simulink model "Appl_PaMemory_CtrlModel"  (R2018b)
settings: configuration reference "CodeConfig_10_ms" (kept outside this file)
undefined symbols (not defined in the file): CAL_PaMem_100MS, CAL_PaMem_90MS, D_ToleranceDistance, FALSE, TRUE
libraries: DareLib x89, simulink x1
(part 2 of 3)

== system Appl_PaMemory_CtrlModel/UpDataInputInfo/InputSignalProcess/HmiMessageDeal ==
  PaMem_IVI_FRSeatMemSet1 : Inport
  PaMem_IVI_FRSeatMemSet2 : Inport  Port=2
  PaMem_IVI_FRSeatMemSet3 : Inport  Port=3
  HmiDeal : Stateflow chart  TreatAsAtomicUnit=on
  SeatMemBtn : Outport
  wires:
  PaMem_IVI_FRSeatMemSet1/1 -> HmiDeal/1(PaMem_IVI_FLSeatMemSet1)
  PaMem_IVI_FRSeatMemSet2/1 -> HmiDeal/2(PaMem_IVI_FLSeatMemSet2)
  HmiDeal/1(SeatMemBtn) -> SeatMemBtn/1
  PaMem_IVI_FRSeatMemSet3/1 -> HmiDeal/3(PaMem_IVI_FLSeatMemSet3)

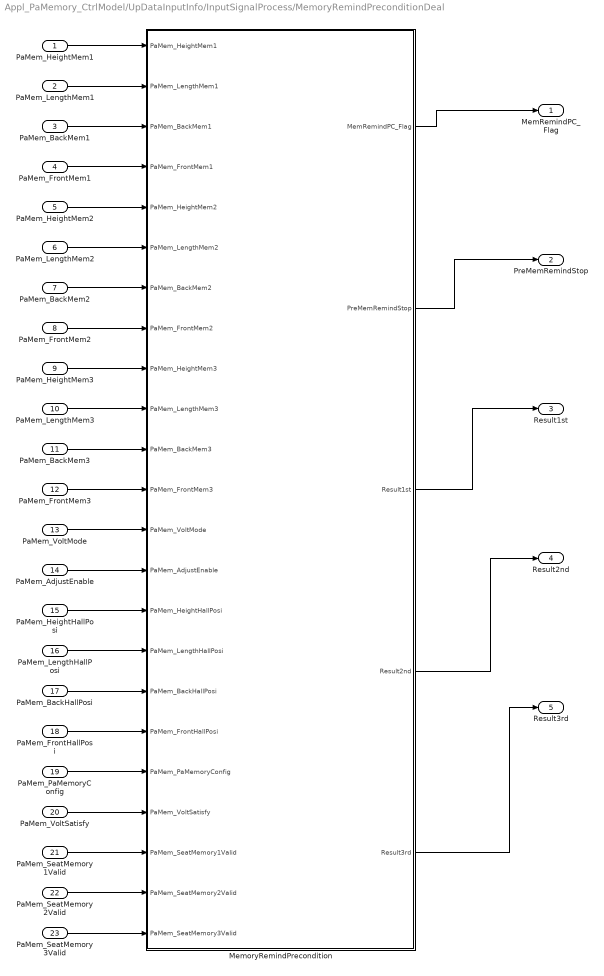
== system Appl_PaMemory_CtrlModel/UpDataInputInfo/InputSignalProcess/MemoryRemindPreconditionDeal ==
  PaMem_HeightMem1 : Inport
  PaMem_LengthMem1 : Inport  Port=2
  PaMem_BackMem1 : Inport  Port=3
  PaMem_FrontMem1 : Inport  Port=4
  PaMem_HeightMem2 : Inport  Port=5
  PaMem_LengthMem2 : Inport  Port=6
  PaMem_BackMem2 : Inport  Port=7
  PaMem_FrontMem2 : Inport  Port=8
  PaMem_HeightMem3 : Inport  Port=9
  PaMem_LengthMem3 : Inport  Port=10
  PaMem_BackMem3 : Inport  Port=11
  PaMem_FrontMem3 : Inport  Port=12
  PaMem_VoltMode : Inport  Port=13
  PaMem_AdjustEnable : Inport  Port=14
  PaMem_HeightHallPosi : Inport  Port=15
  PaMem_LengthHallPosi : Inport  Port=16
  PaMem_BackHallPosi : Inport  Port=17
  PaMem_FrontHallPosi : Inport  Port=18
  PaMem_PaMemoryConfig : Inport  Port=19
  PaMem_VoltSatisfy : Inport  Port=20
  PaMem_SeatMemory1Valid : Inport  Port=21
  PaMem_SeatMemory2Valid : Inport  Port=22
  PaMem_SeatMemory3Valid : Inport  Port=23
  MemoryRemindPrecondition : Stateflow chart  TreatAsAtomicUnit=on
  MemRemindPC_Flag : Outport
  PreMemRemindStop : Outport  Port=2
  Result1st : Outport  Port=3
  Result2nd : Outport  Port=4
  Result3rd : Outport  Port=5
  wires:
  PaMem_FrontMem3/1 -> MemoryRemindPrecondition/12(PaMem_FrontMem3)
  PaMem_VoltMode/1 -> MemoryRemindPrecondition/13(PaMem_VoltMode)
  PaMem_BackMem3/1 -> MemoryRemindPrecondition/11(PaMem_BackMem3)
  PaMem_LengthMem3/1 -> MemoryRemindPrecondition/10(PaMem_LengthMem3)
  PaMem_HeightMem3/1 -> MemoryRemindPrecondition/9(PaMem_HeightMem3)
  PaMem_FrontMem2/1 -> MemoryRemindPrecondition/8(PaMem_FrontMem2)
  PaMem_BackMem2/1 -> MemoryRemindPrecondition/7(PaMem_BackMem2)
  PaMem_LengthMem2/1 -> MemoryRemindPrecondition/6(PaMem_LengthMem2)
  PaMem_HeightMem2/1 -> MemoryRemindPrecondition/5(PaMem_HeightMem2)
  PaMem_FrontMem1/1 -> MemoryRemindPrecondition/4(PaMem_FrontMem1)
  PaMem_HeightMem1/1 -> MemoryRemindPrecondition/1(PaMem_HeightMem1)
  PaMem_BackMem1/1 -> MemoryRemindPrecondition/3(PaMem_BackMem1)
  PaMem_LengthMem1/1 -> MemoryRemindPrecondition/2(PaMem_LengthMem1)
  PaMem_AdjustEnable/1 -> MemoryRemindPrecondition/14(PaMem_AdjustEnable)
  PaMem_HeightHallPosi/1 -> MemoryRemindPrecondition/15(PaMem_HeightHallPosi)
  PaMem_LengthHallPosi/1 -> MemoryRemindPrecondition/16(PaMem_LengthHallPosi)
  PaMem_BackHallPosi/1 -> MemoryRemindPrecondition/17(PaMem_BackHallPosi)
  PaMem_FrontHallPosi/1 -> MemoryRemindPrecondition/18(PaMem_FrontHallPosi)
  MemoryRemindPrecondition/1(MemRemindPC_Flag) -> MemRemindPC_Flag/1
  MemoryRemindPrecondition/2(PreMemRemindStop) -> PreMemRemindStop/1
  MemoryRemindPrecondition/3(Result1st) -> Result1st/1
  MemoryRemindPrecondition/4(Result2nd) -> Result2nd/1
  MemoryRemindPrecondition/5(Result3rd) -> Result3rd/1
  PaMem_PaMemoryConfig/1 -> MemoryRemindPrecondition/19(PaMem_PaMemoryConfig)
  PaMem_VoltSatisfy/1 -> MemoryRemindPrecondition/20(PaMem_VoltSatisfy)
  PaMem_SeatMemory1Valid/1 -> MemoryRemindPrecondition/21(PaMem_SeatMemory1Valid)
  PaMem_SeatMemory2Valid/1 -> MemoryRemindPrecondition/22(PaMem_SeatMemory2Valid)
  PaMem_SeatMemory3Valid/1 -> MemoryRemindPrecondition/23(PaMem_SeatMemory3Valid)

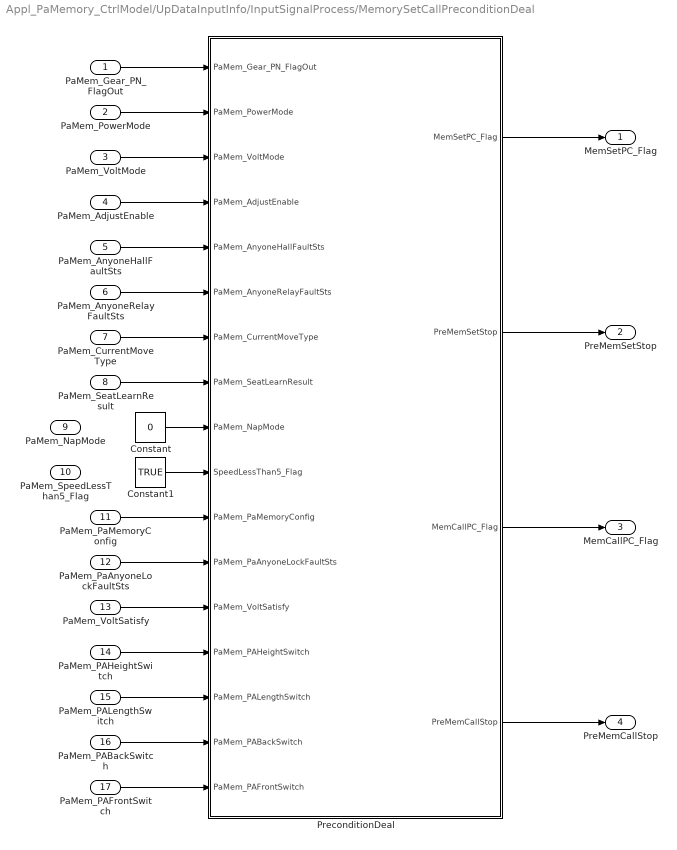
== system Appl_PaMemory_CtrlModel/UpDataInputInfo/InputSignalProcess/MemorySetCallPreconditionDeal ==
  PaMem_Gear_PN_FlagOut : Inport
  PaMem_PowerMode : Inport  Port=2
  PaMem_VoltMode : Inport  Port=3
  PaMem_AdjustEnable : Inport  Port=4
  PaMem_AnyoneHallFaultSts : Inport  Port=5
  PaMem_AnyoneRelayFaultSts : Inport  Port=6
  PaMem_CurrentMoveType : Inport  Port=7
  PaMem_SeatLearnResult : Inport  Port=8
  PaMem_NapMode : Inport  Port=9
  PaMem_SpeedLessThan5_Flag : Inport  Port=10
  PaMem_PaMemoryConfig : Inport  Port=11
  PaMem_PaAnyoneLockFaultSts : Inport  Port=12
  PaMem_VoltSatisfy : Inport  Port=13
  PaMem_PAHeightSwitch : Inport  Port=14
  PaMem_PALengthSwitch : Inport  Port=15
  PaMem_PABackSwitch : Inport  Port=16
  PaMem_PAFrontSwitch : Inport  Port=17
  Constant : Constant  Value=0  OutDataTypeStr=uint8
  Constant1 : Constant  Value=TRUE  OutDataTypeStr=uint8
  PreconditionDeal : Stateflow chart  TreatAsAtomicUnit=on
  MemSetPC_Flag : Outport
  PreMemSetStop : Outport  Port=2
  MemCallPC_Flag : Outport  Port=3
  PreMemCallStop : Outport  Port=4
  wires:
  PaMem_Gear_PN_FlagOut/1 -> PreconditionDeal/1(PaMem_Gear_PN_FlagOut)
  PaMem_PowerMode/1 -> PreconditionDeal/2(PaMem_PowerMode)
  PaMem_VoltMode/1 -> PreconditionDeal/3(PaMem_VoltMode)
  PaMem_AdjustEnable/1 -> PreconditionDeal/4(PaMem_AdjustEnable)
  PaMem_AnyoneHallFaultSts/1 -> PreconditionDeal/5(PaMem_AnyoneHallFaultSts)
  PaMem_CurrentMoveType/1 -> PreconditionDeal/7(PaMem_CurrentMoveType)
  PaMem_SeatLearnResult/1 -> PreconditionDeal/8(PaMem_SeatLearnResult)
  PaMem_AnyoneRelayFaultSts/1 -> PreconditionDeal/6(PaMem_AnyoneRelayFaultSts)
  PreconditionDeal/1(MemSetPC_Flag) -> MemSetPC_Flag/1
  PreconditionDeal/2(PreMemSetStop) -> PreMemSetStop/1
  PreconditionDeal/3(MemCallPC_Flag) -> MemCallPC_Flag/1
  PreconditionDeal/4(PreMemCallStop) -> PreMemCallStop/1
  PaMem_PaMemoryConfig/1 -> PreconditionDeal/11(PaMem_PaMemoryConfig)
  PaMem_PaAnyoneLockFaultSts/1 -> PreconditionDeal/12(PaMem_PaAnyoneLockFaultSts)
  Constant/1 -> PreconditionDeal/9(PaMem_NapMode)
  PaMem_VoltSatisfy/1 -> PreconditionDeal/13(PaMem_VoltSatisfy)
  PaMem_PAHeightSwitch/1 -> PreconditionDeal/14(PaMem_PAHeightSwitch)
  PaMem_PALengthSwitch/1 -> PreconditionDeal/15(PaMem_PALengthSwitch)
  PaMem_PABackSwitch/1 -> PreconditionDeal/16(PaMem_PABackSwitch)
  PaMem_PAFrontSwitch/1 -> PreconditionDeal/17(PaMem_PAFrontSwitch)
  Constant1/1 -> PreconditionDeal/10(SpeedLessThan5_Flag)

== system Appl_PaMemory_CtrlModel/LogicCtrl/LocalAdjustCtrl/MemorySetLogic/FirstPosiMemSetFunc/FirstPosiMemSetFunc/MemoryBack ==
  CurrentB : Inport
  f : TriggerPort  TriggerType=function-call  VariantControl=(inherit)
      settings: CopyFcn=Stateflow.SLINSF.SimulinkMan.removeBlockPreDeleteFcn  PreDeleteFcn=Stateflow.SLINSF.SimulinkMan.unsafePredeleteFcn
  WelcomeRunStatus : DareLib/Dare/setAPI_type  g_funcname=Srvl_SetMemIndexDataU16  g_param=EN_MemIndex_PaMem1_Back  g_type=uint16  g_size=-1
      settings: AttributesFormatString=%<g_funcname>  SourceProductName=Dare Library
  wires:
  CurrentB/1 -> WelcomeRunStatus/1

== system Appl_PaMemory_CtrlModel/LogicCtrl/LocalAdjustCtrl/MemorySetLogic/FirstPosiMemSetFunc/FirstPosiMemSetFunc/MemoryFront ==
  CurrentF : Inport
  f : TriggerPort  TriggerType=function-call  VariantControl=(inherit)
      settings: CopyFcn=Stateflow.SLINSF.SimulinkMan.removeBlockPreDeleteFcn  PreDeleteFcn=Stateflow.SLINSF.SimulinkMan.unsafePredeleteFcn
  WelcomeRunStatus : DareLib/Dare/setAPI_type  g_funcname=Srvl_SetMemIndexDataU16  g_param=EN_MemIndex_PaMem1_Front  g_type=uint16  g_size=-1
      settings: AttributesFormatString=%<g_funcname>  SourceProductName=Dare Library
  wires:
  CurrentF/1 -> WelcomeRunStatus/1

== system Appl_PaMemory_CtrlModel/LogicCtrl/LocalAdjustCtrl/MemorySetLogic/FirstPosiMemSetFunc/FirstPosiMemSetFunc/MemoryHight ==
  CurrentH : Inport
  f : TriggerPort  TriggerType=function-call  VariantControl=(inherit)
      settings: CopyFcn=Stateflow.SLINSF.SimulinkMan.removeBlockPreDeleteFcn  PreDeleteFcn=Stateflow.SLINSF.SimulinkMan.unsafePredeleteFcn
  WelcomeRunStatus : DareLib/Dare/setAPI_type  g_funcname=Srvl_SetMemIndexDataU16  g_param=EN_MemIndex_PaMem1_Height  g_type=uint16  g_size=-1
      settings: AttributesFormatString=%<g_funcname>  SourceProductName=Dare Library
  wires:
  CurrentH/1 -> WelcomeRunStatus/1

== system Appl_PaMemory_CtrlModel/LogicCtrl/LocalAdjustCtrl/MemorySetLogic/FirstPosiMemSetFunc/FirstPosiMemSetFunc/MemoryLength ==
  CurrentL : Inport
  f : TriggerPort  TriggerType=function-call  VariantControl=(inherit)
      settings: CopyFcn=Stateflow.SLINSF.SimulinkMan.removeBlockPreDeleteFcn  PreDeleteFcn=Stateflow.SLINSF.SimulinkMan.unsafePredeleteFcn
  WelcomeRunStatus : DareLib/Dare/setAPI_type  g_funcname=Srvl_SetMemIndexDataU16  g_param=EN_MemIndex_PaMem1_Length  g_type=uint16  g_size=-1
      settings: AttributesFormatString=%<g_funcname>  SourceProductName=Dare Library
  wires:
  CurrentL/1 -> WelcomeRunStatus/1

== system Appl_PaMemory_CtrlModel/LogicCtrl/LocalAdjustCtrl/MemorySetLogic/FirstPosiMemSetFunc/FirstPosiMemSetFunc/MemoryValid ==
  Sts : Inport
  f : TriggerPort  TriggerType=function-call  VariantControl=(inherit)
      settings: CopyFcn=Stateflow.SLINSF.SimulinkMan.removeBlockPreDeleteFcn  PreDeleteFcn=Stateflow.SLINSF.SimulinkMan.unsafePredeleteFcn
  WelcomeRunStatus : DareLib/Dare/setAPI_type  g_funcname=Srvl_SetMemIndexDataU8  g_param=EN_MemIndex_PaMem1_ValidFlag  g_type=uint16  g_size=-1
      settings: AttributesFormatString=%<g_funcname>  SourceProductName=Dare Library
  wires:
  Sts/1 -> WelcomeRunStatus/1

== system Appl_PaMemory_CtrlModel/LogicCtrl/LocalAdjustCtrl/MemorySetLogic/SecondPosiMemSetFunc/SecondPosiMemSetFunc/MemoryBack ==
  CurrentB : Inport
  f : TriggerPort  TriggerType=function-call  VariantControl=(inherit)
      settings: CopyFcn=Stateflow.SLINSF.SimulinkMan.removeBlockPreDeleteFcn  PreDeleteFcn=Stateflow.SLINSF.SimulinkMan.unsafePredeleteFcn
  WelcomeRunStatus : DareLib/Dare/setAPI_type  g_funcname=Srvl_SetMemIndexDataU16  g_param=EN_MemIndex_PaMem2_Back  g_type=uint16  g_size=-1
      settings: AttributesFormatString=%<g_funcname>  SourceProductName=Dare Library
  wires:
  CurrentB/1 -> WelcomeRunStatus/1

== system Appl_PaMemory_CtrlModel/LogicCtrl/LocalAdjustCtrl/MemorySetLogic/SecondPosiMemSetFunc/SecondPosiMemSetFunc/MemoryFront ==
  CurrentF : Inport
  f : TriggerPort  TriggerType=function-call  VariantControl=(inherit)
      settings: CopyFcn=Stateflow.SLINSF.SimulinkMan.removeBlockPreDeleteFcn  PreDeleteFcn=Stateflow.SLINSF.SimulinkMan.unsafePredeleteFcn
  WelcomeRunStatus : DareLib/Dare/setAPI_type  g_funcname=Srvl_SetMemIndexDataU16  g_param=EN_MemIndex_PaMem2_Front  g_type=uint16  g_size=-1
      settings: AttributesFormatString=%<g_funcname>  SourceProductName=Dare Library
  wires:
  CurrentF/1 -> WelcomeRunStatus/1

== system Appl_PaMemory_CtrlModel/LogicCtrl/LocalAdjustCtrl/MemorySetLogic/SecondPosiMemSetFunc/SecondPosiMemSetFunc/MemoryHight ==
  CurrentH : Inport
  f : TriggerPort  TriggerType=function-call  VariantControl=(inherit)
      settings: CopyFcn=Stateflow.SLINSF.SimulinkMan.removeBlockPreDeleteFcn  PreDeleteFcn=Stateflow.SLINSF.SimulinkMan.unsafePredeleteFcn
  WelcomeRunStatus : DareLib/Dare/setAPI_type  g_funcname=Srvl_SetMemIndexDataU16  g_param=EN_MemIndex_PaMem2_Height  g_type=uint16  g_size=-1
      settings: AttributesFormatString=%<g_funcname>  SourceProductName=Dare Library
  wires:
  CurrentH/1 -> WelcomeRunStatus/1

== system Appl_PaMemory_CtrlModel/LogicCtrl/LocalAdjustCtrl/MemorySetLogic/SecondPosiMemSetFunc/SecondPosiMemSetFunc/MemoryLength ==
  CurrentL : Inport
  f : TriggerPort  TriggerType=function-call  VariantControl=(inherit)
      settings: CopyFcn=Stateflow.SLINSF.SimulinkMan.removeBlockPreDeleteFcn  PreDeleteFcn=Stateflow.SLINSF.SimulinkMan.unsafePredeleteFcn
  WelcomeRunStatus : DareLib/Dare/setAPI_type  g_funcname=Srvl_SetMemIndexDataU16  g_param=EN_MemIndex_PaMem2_Length  g_type=uint16  g_size=-1
      settings: AttributesFormatString=%<g_funcname>  SourceProductName=Dare Library
  wires:
  CurrentL/1 -> WelcomeRunStatus/1

== system Appl_PaMemory_CtrlModel/LogicCtrl/LocalAdjustCtrl/MemorySetLogic/SecondPosiMemSetFunc/SecondPosiMemSetFunc/MemoryValid ==
  Sts : Inport
  f : TriggerPort  TriggerType=function-call  VariantControl=(inherit)
      settings: CopyFcn=Stateflow.SLINSF.SimulinkMan.removeBlockPreDeleteFcn  PreDeleteFcn=Stateflow.SLINSF.SimulinkMan.unsafePredeleteFcn
  WelcomeRunStatus : DareLib/Dare/setAPI_type  g_funcname=Srvl_SetMemIndexDataU8  g_param=EN_MemIndex_PaMem2_ValidFlag  g_type=uint16  g_size=-1
      settings: AttributesFormatString=%<g_funcname>  SourceProductName=Dare Library
  wires:
  Sts/1 -> WelcomeRunStatus/1

== system Appl_PaMemory_CtrlModel/LogicCtrl/LocalAdjustCtrl/MemorySetLogic/ThirdPosiMemSetFunc/ThirdPosiMemSetFunc/MemoryBack ==
  CurrentB : Inport
  f : TriggerPort  TriggerType=function-call  VariantControl=(inherit)
      settings: CopyFcn=Stateflow.SLINSF.SimulinkMan.removeBlockPreDeleteFcn  PreDeleteFcn=Stateflow.SLINSF.SimulinkMan.unsafePredeleteFcn
  WelcomeRunStatus : DareLib/Dare/setAPI_type  g_funcname=Srvl_SetMemIndexDataU16  g_param=EN_MemIndex_PaMem3_Back  g_type=uint16  g_size=-1
      settings: AttributesFormatString=%<g_funcname>  SourceProductName=Dare Library
  wires:
  CurrentB/1 -> WelcomeRunStatus/1

== system Appl_PaMemory_CtrlModel/LogicCtrl/LocalAdjustCtrl/MemorySetLogic/ThirdPosiMemSetFunc/ThirdPosiMemSetFunc/MemoryFront ==
  CurrentF : Inport
  f : TriggerPort  TriggerType=function-call  VariantControl=(inherit)
      settings: CopyFcn=Stateflow.SLINSF.SimulinkMan.removeBlockPreDeleteFcn  PreDeleteFcn=Stateflow.SLINSF.SimulinkMan.unsafePredeleteFcn
  WelcomeRunStatus : DareLib/Dare/setAPI_type  g_funcname=Srvl_SetMemIndexDataU16  g_param=EN_MemIndex_PaMem3_Front  g_type=uint16  g_size=-1
      settings: AttributesFormatString=%<g_funcname>  SourceProductName=Dare Library
  wires:
  CurrentF/1 -> WelcomeRunStatus/1

== system Appl_PaMemory_CtrlModel/LogicCtrl/LocalAdjustCtrl/MemorySetLogic/ThirdPosiMemSetFunc/ThirdPosiMemSetFunc/MemoryHight ==
  CurrentH : Inport
  f : TriggerPort  TriggerType=function-call  VariantControl=(inherit)
      settings: CopyFcn=Stateflow.SLINSF.SimulinkMan.removeBlockPreDeleteFcn  PreDeleteFcn=Stateflow.SLINSF.SimulinkMan.unsafePredeleteFcn
  WelcomeRunStatus : DareLib/Dare/setAPI_type  g_funcname=Srvl_SetMemIndexDataU16  g_param=EN_MemIndex_PaMem3_Height  g_type=uint16  g_size=-1
      settings: AttributesFormatString=%<g_funcname>  SourceProductName=Dare Library
  wires:
  CurrentH/1 -> WelcomeRunStatus/1

== system Appl_PaMemory_CtrlModel/LogicCtrl/LocalAdjustCtrl/MemorySetLogic/ThirdPosiMemSetFunc/ThirdPosiMemSetFunc/MemoryLength ==
  CurrentL : Inport
  f : TriggerPort  TriggerType=function-call  VariantControl=(inherit)
      settings: CopyFcn=Stateflow.SLINSF.SimulinkMan.removeBlockPreDeleteFcn  PreDeleteFcn=Stateflow.SLINSF.SimulinkMan.unsafePredeleteFcn
  WelcomeRunStatus : DareLib/Dare/setAPI_type  g_funcname=Srvl_SetMemIndexDataU16  g_param=EN_MemIndex_PaMem3_Length  g_type=uint16  g_size=-1
      settings: AttributesFormatString=%<g_funcname>  SourceProductName=Dare Library
  wires:
  CurrentL/1 -> WelcomeRunStatus/1

== system Appl_PaMemory_CtrlModel/LogicCtrl/LocalAdjustCtrl/MemorySetLogic/ThirdPosiMemSetFunc/ThirdPosiMemSetFunc/MemoryValid ==
  Sts : Inport
  f : TriggerPort  TriggerType=function-call  VariantControl=(inherit)
      settings: CopyFcn=Stateflow.SLINSF.SimulinkMan.removeBlockPreDeleteFcn  PreDeleteFcn=Stateflow.SLINSF.SimulinkMan.unsafePredeleteFcn
  WelcomeRunStatus : DareLib/Dare/setAPI_type  g_funcname=Srvl_SetMemIndexDataU8  g_param=EN_MemIndex_PaMem3_ValidFlag  g_type=uint16  g_size=-1
      settings: AttributesFormatString=%<g_funcname>  SourceProductName=Dare Library
  wires:
  Sts/1 -> WelcomeRunStatus/1

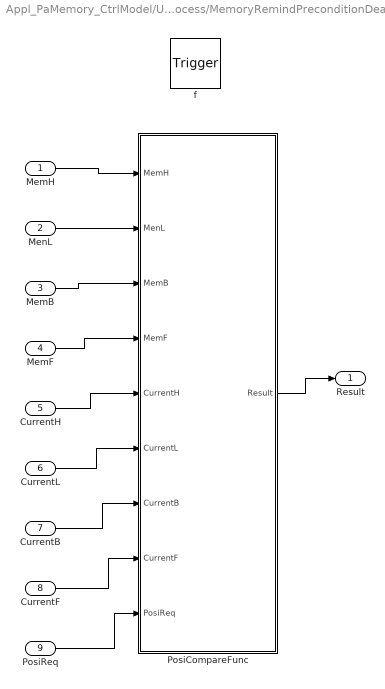
== system Appl_PaMemory_CtrlModel/UpDataInputInfo/InputSignalProcess/MemoryRemindPreconditionDeal/MemoryRemindPrecondition/PosiCompareFunc ==
  MemH : Inport
  MenL : Inport  Port=2
  MemB : Inport  Port=3
  MemF : Inport  Port=4
  CurrentH : Inport  Port=5
  CurrentL : Inport  Port=6
  CurrentB : Inport  Port=7
  CurrentF : Inport  Port=8
  PosiReq : Inport  Port=9
  f : TriggerPort  TriggerType=function-call  VariantControl=(inherit)
      settings: CopyFcn=Stateflow.SLINSF.SimulinkMan.removeBlockPreDeleteFcn  PreDeleteFcn=Stateflow.SLINSF.SimulinkMan.unsafePredeleteFcn
  PosiCompareFunc : Stateflow chart  TreatAsAtomicUnit=on
  "Result " : Outport
  wires:
  MemB/1 -> PosiCompareFunc/3(MemB)
  MemF/1 -> PosiCompareFunc/4(MemF)
  CurrentH/1 -> PosiCompareFunc/5(CurrentH)
  MenL/1 -> PosiCompareFunc/2(MenL)
  CurrentL/1 -> PosiCompareFunc/6(CurrentL)
  MemH/1 -> PosiCompareFunc/1(MemH)
  CurrentB/1 -> PosiCompareFunc/7(CurrentB)
  CurrentF/1 -> PosiCompareFunc/8(CurrentF)
  PosiCompareFunc/1(Result) -> "Result "/1
  PosiReq/1 -> PosiCompareFunc/9(PosiReq)

== stateflow chart Appl_PaMemory_CtrlModel/UpDataInputInfo/InputSignalProcess/CallMemDeal/CallMemory ==
  state NoneMemoryCall
    en:
    MemoryHeightPosi = 0;
    MemoryLengthPosi = 0;
    MemoryBackPosi = 0;
    MemoryFrontPosi = 0;
    MemoryValid = FALSE;
  state AcquireMemory2ndPosi
    en:
    MemoryHeightPosi = PaMem_HeightMem2;
    MemoryLengthPosi = PaMem_LengthMem2;
    MemoryBackPosi = PaMem_BackMem2;
    MemoryFrontPosi = PaMem_FrontMem2;
    MemoryValid = PaMem_SeatMemory2Valid;
  state AcquireMemory1stPosi
    en:
    MemoryHeightPosi = PaMem_HeightMem1;
    MemoryLengthPosi = PaMem_LengthMem1;
    MemoryBackPosi = PaMem_BackMem1;
    MemoryFrontPosi = PaMem_FrontMem1;
    MemoryValid = PaMem_SeatMemory1Valid;
  state AcquireMemory3rdPosi
    en:
    MemoryHeightPosi = PaMem_HeightMem3;
    MemoryLengthPosi = PaMem_LengthMem3;
    MemoryBackPosi = PaMem_BackMem3;
    MemoryFrontPosi = PaMem_FrontMem3;
    MemoryValid = PaMem_SeatMemory3Valid;
  (default) -> NoneMemoryCall
  NoneMemoryCall -> AcquireMemory1stPosi [order 1] : /* 调用位置1 */
      | [SeatMemBtn == enMemBtn.EN_MemBtn_Call1]
  AcquireMemory1stPosi -> NoneMemoryCall [order 1] : /* 无调用 */
      | [SeatMemBtn != enMemBtn.EN_MemBtn_Call1 ...
      | && SeatMemBtn != enMemBtn.EN_MemBtn_Call2 ...
      | && SeatMemBtn != enMemBtn.EN_MemBtn_Call3]
  NoneMemoryCall -> AcquireMemory2ndPosi [order 2] : /* 调用位置2 */
      | [SeatMemBtn == enMemBtn.EN_MemBtn_Call2]
  AcquireMemory2ndPosi -> NoneMemoryCall [order 1] : /* 无调用 */
      | [SeatMemBtn != enMemBtn.EN_MemBtn_Call1 ...
      | && SeatMemBtn != enMemBtn.EN_MemBtn_Call2 ...
      | && SeatMemBtn != enMemBtn.EN_MemBtn_Call3]
  NoneMemoryCall -> AcquireMemory3rdPosi [order 3] : /* 调用位置3 */
      | [SeatMemBtn == enMemBtn.EN_MemBtn_Call3]
  AcquireMemory3rdPosi -> NoneMemoryCall [order 1] : /* 无调用 */
      | [SeatMemBtn != enMemBtn.EN_MemBtn_Call1 ...
      | && SeatMemBtn != enMemBtn.EN_MemBtn_Call2 ...
      | && SeatMemBtn != enMemBtn.EN_MemBtn_Call3]
  AcquireMemory1stPosi -> AcquireMemory2ndPosi [order 3] : /* 调用位置2 */
      | [SeatMemBtn == enMemBtn.EN_MemBtn_Call2]
  AcquireMemory3rdPosi -> AcquireMemory2ndPosi [order 3] : /* 调用位置2 */
      | [SeatMemBtn == enMemBtn.EN_MemBtn_Call2]
  AcquireMemory2ndPosi -> AcquireMemory3rdPosi [order 3] : /* 调用位置3 */
      | [SeatMemBtn == enMemBtn.EN_MemBtn_Call3]
  AcquireMemory2ndPosi -> AcquireMemory1stPosi [order 2] : /* 调用位置1 */
      | [SeatMemBtn == enMemBtn.EN_MemBtn_Call1]
  AcquireMemory1stPosi -> AcquireMemory3rdPosi [order 2] : /* 调用位置3 */
      | [SeatMemBtn == enMemBtn.EN_MemBtn_Call3]
  AcquireMemory3rdPosi -> AcquireMemory1stPosi [order 2] : /* 调用位置1 */
      | [SeatMemBtn == enMemBtn.EN_MemBtn_Call1]
  data: PaMem_HeightMem1 input; MemoryHeightPosi output uint16; MemoryLengthPosi output uint16; MemoryBackPosi output uint16; MemoryFrontPosi output uint16; MemoryValid output uint8; PaMem_LengthMem1 input; PaMem_BackMem1 input; PaMem_FrontMem1 input; PaMem_HeightMem2 input; PaMem_LengthMem2 input; PaMem_BackMem2 input; PaMem_FrontMem2 input; PaMem_HeightMem3 input; PaMem_LengthMem3 input; PaMem_BackMem3 input; PaMem_FrontMem3 input; SeatMemBtn input; TRUE parameter; FALSE parameter; PaMem_SeatMemory1Valid input; PaMem_SeatMemory2Valid input; PaMem_SeatMemory3Valid input

== stateflow chart Appl_PaMemory_CtrlModel/UpDataInputInfo/InputSignalProcess/MemoryRemindPreconditionDeal/MemoryRemindPrecondition ==
  state Result = PosiCompareFunc(MemH,MenL,MemB,MemF,CurrentH,CurrentL,CurrentB,CurrentF,PosiReq) [function]
  state CompareCurrentAndMemoryPosi [parallel]
    du:
    Result1st = PosiCompareFunc(0,PaMem_LengthMem1,PaMem_BackMem1,0,0,PaMem_LengthHallPosi,PaMem_BackHallPosi,0,PaMem_SeatMemory1Valid);
    Result2nd = PosiCompareFunc(0,PaMem_LengthMem2,PaMem_BackMem2,0,0,PaMem_LengthHallPosi,PaMem_BackHallPosi,0,PaMem_SeatMemory2Valid);
    Result3rd = PosiCompareFunc(0,PaMem_LengthMem3,PaMem_BackMem3,0,0,PaMem_LengthHallPosi,PaMem_BackHallPosi,0,PaMem_SeatMemory3Valid);
    settings: executionOrder=1
  state MemoryRemindPreconditionDeal [parallel]
    settings: executionOrder=2
    state PreconditionNotSatisfied
      en:
      MemRemindPC_Flag = FALSE;
    state PreconditionSatisfied
      en:
      MemRemindPC_Flag = TRUE;
    (default) -> PreconditionNotSatisfied
    PreconditionNotSatisfied -> PreconditionSatisfied : /*记忆功能使能 == 0x1:TRUE
        | && 记忆提示功能使能 == 0x1:Enable
        | && 电压模式 == 正常
        | /PreMemRemindStop = 0x0:enNone;*/
        | [PaMem_AdjustEnable == TRUE ...
        | && PaMem_PaMemoryConfig == TRUE ...
        | && PaMem_VoltSatisfy == TRUE ...
        | && PaMem_VoltMode == enFinalPowerMode.EN_NORMAL_VOLT]
        | /PreMemRemindStop = enMemStopCause.EN_MemStop_NULL;
    PreconditionSatisfied -> PreconditionNotSatisfied [order 1] : /*F101记忆功能 != 0x1:TRUE
        | || 记忆提示功能配置 != 0x1:Enable
        | /PreMemRemindStop = 0xA:enConfigError;*/
        | [PaMem_AdjustEnable != TRUE || PaMem_PaMemoryConfig != TRUE]
        | /PreMemRemindStop = enMemStopCause.EN_MemStop_ConfigError;
    PreconditionSatisfied -> PreconditionNotSatisfied [order 2] : /*电压模式 != 正常
        | /PreMemRemindStop = 0xE:enVoltageError;*/
        | [PaMem_VoltMode != enFinalPowerMode.EN_NORMAL_VOLT ...
        | || PaMem_VoltSatisfy != TRUE]
        | /PreMemRemindStop = enMemStopCause.EN_MemStop_VoltageErr;
  data: MemH function_input; MenL function_input; MemB function_input; MemF function_input; CurrentH function_input; CurrentL function_input; CurrentB function_input; CurrentF function_input; Result function_output; PosiReq function_input; PaMem_HeightMem1 input; PaMem_LengthMem1 input; PaMem_BackMem1 input; PaMem_FrontMem1 input; PaMem_HeightMem2 input; PaMem_LengthMem2 input; PaMem_BackMem2 input; PaMem_FrontMem2 input; PaMem_HeightMem3 input; PaMem_LengthMem3 input; PaMem_BackMem3 input; PaMem_FrontMem3 input; PaMem_VoltMode input; TRUE parameter; PaMem_AdjustEnable input; FALSE parameter; MemRemindPC_Flag output uint8; PreMemRemindStop output Enum: enMemStopCause; Result1st output uint8; Result2nd output uint8; Result3rd output uint8; PaMem_HeightHallPosi input; PaMem_LengthHallPosi input; PaMem_BackHallPosi input; PaMem_FrontHallPosi input; PaMem_PaMemoryConfig input; PaMem_VoltSatisfy input; PaMem_SeatMemory1Valid input; PaMem_SeatMemory2Valid input; PaMem_SeatMemory3Valid input

== stateflow chart Appl_PaMemory_CtrlModel/LogicCtrl/LocalAdjustCtrl/MemorySetLogic ==
  state FirstPosiMemSetFunc(SeatMemCfg,CurrentH,CurrentL,CurrentB,CurrentF) [function]
  state MemorySetInactive
    en:
    FRSeatMemSetSts = enMemSetFb.EN_MemSetFb_NULL;
    MsgSendFinishedFlag = FALSE;
  state SecondPosiMemSetFunc(SeatMemCfg,CurrentH,CurrentL,CurrentB,CurrentF) [function]
  state MemorySetActive
    state Wait
      (default) -> (junction 127)
      Wait -> (junction 127) [order 1]
      (junction 127) -> (junction 30)
      (junction 30) -> (junction 122) [order 1] : /*初始前置条件不符合*/
          | [MemSetPC_Flag == FALSE]
      (junction 30) -> (junction 33) [order 2]
      (junction 122) -> (junction 124) : {WaitTimer = 0;}
      (junction 33) -> (junction 35) [order 1] : /*记忆设置1*/
          | [SeatMemBtn == enMemBtn.EN_MemBtn_Set1]
      (junction 33) -> (junction 39) [order 2]
      (junction 35) -> (junction 37) : {FRTempSeatMemSetSts = enMemSetFb.EN_MemSetFb_S1;
          | FirstPosiMemSetFunc(PaMem_AdjustEnable,PaMem_HeightHallPosi,PaMem_LengthHallPosi,PaMem_BackHallPosi,PaMem_FrontHallPosi);}
      (junction 37) -> (junction 39)
      (junction 39) -> (junction 42)
      (junction 42) -> (junction 44) [order 1] : /*记忆设置2*/
          | [SeatMemBtn == enMemBtn.EN_MemBtn_Set2]
      (junction 42) -> (junction 48) [order 2]
      (junction 44) -> (junction 46) : {FRTempSeatMemSetSts = enMemSetFb.EN_MemSetFb_S2;
          | SecondPosiMemSetFunc(PaMem_AdjustEnable,PaMem_HeightHallPosi,PaMem_LengthHallPosi,PaMem_BackHallPosi,PaMem_FrontHallPosi);}
      (junction 46) -> (junction 48)
      (junction 48) -> (junction 51)
      (junction 51) -> (junction 53) [order 1] : /*记忆设置3*/
          | [SeatMemBtn == enMemBtn.EN_MemBtn_Set3]
      (junction 51) -> (junction 57) [order 2]
      (junction 53) -> (junction 55) : {FRTempSeatMemSetSts = enMemSetFb.EN_MemSetFb_S3;
          | ThirdPosiMemSetFunc(PaMem_AdjustEnable,PaMem_HeightHallPosi,PaMem_LengthHallPosi,PaMem_BackHallPosi,PaMem_FrontHallPosi);}
      (junction 55) -> (junction 57)
      (junction 57) -> (junction 60) : {FRSeatMemSetSts = enMemSetFb.EN_MemSetFb_NULL;}
      (junction 60) -> (junction 62)
      (junction 62) -> (junction 64) [order 1] : /*使用延时代替EEPROM操作结果*/
          | [WaitTimer < CAL_PaMem_100MS]
      (junction 62) -> (junction 68) [order 2] : {WaitTimer = CAL_PaMem_100MS;}
      (junction 64) -> (junction 66) : {WaitTimer++ ;}
      (junction 66) -> (junction 68)
      (junction 124) -> (junction 66)
      (junction 68) -> (junction 72)
    state Succeed
      en:
      FRSeatMemSetSts = FRTempSeatMemSetSts;
      WaitTimer = 0;
      WaitTimeCnt = 0;
      SetCanSendMemStsAndMsg(FRSeatMemSetSts);
      SetCanSendEvent(0x3B2);
      du:
      WaitTimeCnt += 1;
    state Fail
      en:
      FRSeatMemSetSts = enMemSetFb.EN_MemSetFb_Fail;
      WaitTimer = 0;
      WaitTimeCnt = 0;
      SetCanSendMemStsAndMsg(FRSeatMemSetSts);
      SetCanSendEvent(0x3B2);
      du:
      WaitTimeCnt += 1;
    note: /*如果服务层没有CAN反馈标志，使用延时90ms(20ms/5帧)*/
    state MessageSendFinish
      en:
      MsgSendFinishedFlag = TRUE;
      FRSeatMemSetSts = enMemSetFb.EN_MemSetFb_NULL;
    (default) -> Wait
    Wait -> Succeed [order 2] : /*存储结束*/
        | [WaitTimer >= CAL_PaMem_100MS]
    Wait -> Fail [order 1] : /*前置条件不符合*/
        | [MemSetPC_Flag == FALSE]
        | /MemSetStopReason = PreMemSetStop;
    Wait -> Fail [commented out] : /*记忆存储失败，如果无此接口，删除*/
    Succeed -> MessageSendFinish : /*Srvl_CAN反馈报文发送完成 || 延时90ms*/
        | [WaitTimeCnt >= CAL_PaMem_90MS || GetCanSendEvent() == TRUE]
    Fail -> MessageSendFinish : /*Srvl_CAN反馈报文发送完成 || 延时90ms*/
        | [WaitTimeCnt >= CAL_PaMem_90MS || GetCanSendEvent() == TRUE]
  state ThirdPosiMemSetFunc(SeatMemCfg,CurrentH,CurrentL,CurrentB,CurrentF) [function]
  state SetCanSendEvent(In1) [function]
  state Out1 = GetCanSendEvent [function]
  state SetCanSendMemStsAndMsg(In1) [function]
  (default) -> MemorySetInactive
  MemorySetInactive -> MemorySetActive [order 1] : /*SeatMemBtn变为MemorizeButton1*/
      | [hasChangedTo(SeatMemBtn,enMemBtn.EN_MemBtn_Set1)]
  MemorySetInactive -> MemorySetActive [order 2] : /*SeatMemBtn变为MemorizeButton2*/
      | [hasChangedTo(SeatMemBtn,enMemBtn.EN_MemBtn_Set2)]
  MemorySetInactive -> MemorySetActive [order 3] : /*SeatMemBtn变为MemorizeButton3*/
      | [hasChangedTo(SeatMemBtn,enMemBtn.EN_MemBtn_Set3)]
  MemorySetActive -> MemorySetInactive : [MsgSendFinishedFlag == TRUE]
  data: SeatMemCfg function_input; CurrentH function_input; CurrentL function_input; CurrentB function_input; CurrentF function_input; SeatMemCfg function_input; CurrentH function_input; CurrentL function_input; CurrentB function_input; CurrentF function_input; SeatMemCfg function_input; CurrentH function_input; CurrentL function_input; CurrentB function_input; CurrentF function_input; In1 function_input; Out1 function_output; In1 function_input; FRSeatMemSetSts output Enum: enMemSetFb; MsgSendFinishedFlag local uint8; TRUE parameter; FALSE parameter; SeatMemBtn input; PaMem_HeightHallPosi input; PaMem_LengthHallPosi input; PaMem_BackHallPosi input; PaMem_FrontHallPosi input; MemSetPC_Flag input; WaitTimer local uint8; CAL_PaMem_100MS parameter; PreMemSetStop input; MemSetStopReason output Enum: enMemStopCause; FRTempSeatMemSetSts local Enum: enMemSetFb; PaMem_AdjustEnable input; CAL_PaMem_90MS parameter; WaitTimeCnt local uint16

== stateflow chart Appl_PaMemory_CtrlModel/UpDataInputInfo/InputSignalProcess/MemoryRemindPreconditionDeal/MemoryRemindPrecondition/PosiCompareFunc/PosiCompareFunc ==
  (default) -> (junction 15)
  (junction 15) -> (junction 30) [order 1] : /* 没有记忆位置 */
      | [PosiReq == FALSE]
  (junction 15) -> (junction 17) [order 2]
  (junction 30) -> (junction 34) : {Result = 2;}
  (junction 17) -> (junction 19) [order 1] : /* 当前位置在记忆位置范围内 */
      | [CurrentH <= MemH + D_ToleranceDistance ...
      | && MemH <= CurrentH  + D_ToleranceDistance ...
      | && CurrentL <= MenL + D_ToleranceDistance ...
      | && MenL <= CurrentL  + D_ToleranceDistance ...
      | && CurrentB <= MemB + D_ToleranceDistance ...
      | && MemB <= CurrentB  + D_ToleranceDistance ...
      | && CurrentF <= MemF + D_ToleranceDistance ...
      | && MemF <= CurrentF  + D_ToleranceDistance]
  (junction 17) -> (junction 23) [order 2] : {Result = FALSE;}
  (junction 19) -> (junction 21) : {Result = TRUE;}
  (junction 21) -> (junction 23)
  (junction 34) -> (junction 21)
  (junction 23) -> (junction 26)
  data: MemH input uint16; MenL input uint16; MemB input uint16; MemF input uint16; CurrentH input uint16; CurrentL input uint16; CurrentB input uint16; CurrentF input uint16; Result output uint8; TRUE parameter; FALSE parameter; D_ToleranceDistance parameter; PosiReq input uint8

== stateflow chart Appl_PaMemory_CtrlModel/LogicCtrl/LocalAdjustCtrl/MemoryRemindLogic ==
  state SetCanSendEvent(In1) [function]
  state SetCanSendFRSeatPosMsg(In1) [function]
  state Out1 = GetCanSendEvent [function]
  state WriteFLSeatPosMsg(Sts) [function]
  state Init [commented out]
    en:
    FirstTimeCnt = 0;
    du:
    FirstTimeCnt += 1;
  state PositionNoChange [commented out]
    en:
    FRSeatPosMsg = FALSE;
    WriteFLSeatPosMsg(FRSeatPosMsg);
  state PositionNoChange1
    en:
    FRSeatPosMsg = FALSE;
  state PositionChange [commented out]
    en:
    FRSeatPosMsg = TRUE;
    WriteFLSeatPosMsg(FRSeatPosMsg);
  note: ?
  state PositionChange1
    en:
    FRSeatPosMsg = TRUE;
    SetCanSendFRSeatPosMsg(FRSeatPosMsg);
    SetCanSendEvent(0x3B2);
  (default) -> Init [commented out]
  Init -> (junction 3) [commented out] : /* 上电获取eeprom延时 */
      | [FirstTimeCnt > CAL_PaMem_90MS]
  (junction 3) -> PositionNoChange [commented out]
  (junction 3) -> PositionChange [commented out] : /*FLSeatPosMsg存储的
      | EEPROM数据 == 0x1:enChange*/
      | [PaMem_FLSeatPosMsg == TRUE]
  (default) -> PositionNoChange1
  PositionNoChange -> PositionChange [commented out] : /*满足【前置条件】&&【触发条件1】
      | 运动类型由手动调节变为静止
      | && MemRemindPC_Flag == TRUE
      | &&(Result1st != TRUE
      | || Result2nd != TRUE
      | || Result3rd != TRUE)*/
      | [hasChangedFrom(PaMem_CurrentMoveType, ...
      | enSeatMotorRunType.EN_ManualEnable) ...
      | && PaMem_CurrentMoveType == enSeatMotorRunType.EN_NULL ...
      | && MemRemindPC_Flag == TRUE ...
      | &&(Result1st != TRUE ...
      | && Result2nd != TRUE ...
      | && Result3rd != TRUE)]
  PositionChange -> PositionNoChange [commented out] : /*恢复出厂标志位 == TRUE */
      | [PaMem_GetRecoverDefaultFlag == TRUE]
  PositionChange -> PositionNoChange [commented out] : /*满足【前置条件】||【触发条件2】
      | (Result1st == TRUE
      | || Result2nd == TRUE
      | || Result3rd == TRUE)
      | || MemRemindPC_Flag == FALSE*/
      | [(Result1st == TRUE ...
      | || Result2nd == TRUE ...
      | || Result3rd == TRUE) ...
      | || MemRemindPC_Flag == FALSE]
  PositionNoChange1 -> PositionChange1 : /*满足【前置条件】&&【触发条件1】
      | 运动类型由手动调节变为静止
      | && MemRemindPC_Flag == TRUE
      | &&(Result1st != TRUE
      | || Result2nd != TRUE
      | || Result3rd != TRUE)*/
      | [hasChangedFrom(PaMem_CurrentMoveType, ...
      | enSeatMotorRunType.EN_ManualEnable) ...
      | && PaMem_CurrentMoveType == enSeatMotorRunType.EN_NULL ...
      | && MemRemindPC_Flag == TRUE ...
      | && (Result1st != 2 || Result2nd != 2 || Result3rd != 2) ...
      | && Result1st != TRUE ...
      | && Result2nd != TRUE ...
      | && Result3rd != TRUE ]
  PositionChange1 -> PositionNoChange1 [order 1] : /*恢复出厂标志位 == TRUE */
      | [PaMem_GetRecoverDefaultFlag == TRUE ...
      | || MemRemindPC_Flag == FALSE]
  PositionChange1 -> PositionNoChange1 [order 2] : /*超时时间*/
      | [GetCanSendEvent() == TRUE]
  data: In1 function_input; In1 function_input; Out1 function_output; Sts function_input; FRSeatPosMsg output uint8; TRUE parameter; FALSE parameter; PaMem_FLSeatPosMsg input; MemRemindPC_Flag input; Result1st input; Result2nd input; Result3rd input; PaMem_CurrentMoveType input; PaMem_GetRecoverDefaultFlag input; FirstTimeCnt local uint8; CAL_PaMem_90MS parameter

== stateflow chart Appl_PaMemory_CtrlModel/UpDataInputInfo/InputSignalProcess/HmiMessageDeal/HmiDeal ==
  state MemoryMessageConflictDeal [parallel]
    settings: executionOrder=1
    (default) -> (junction 241)
    MemoryMessageConflictDeal -> (junction 241)
    (junction 241) -> (junction 232) : {ActionCnt = 0;}
    (junction 232) -> (junction 233) [order 1] : /* 调用1 */
        | [PaMem_IVI_FLSeatMemSet1 > enMemSet.EN_MemSet_NULL ...
        | && PaMem_IVI_FLSeatMemSet1 < enMemSet.EN_MemSet_Clean]
    (junction 232) -> (junction 234) [order 2]
    (junction 233) -> (junction 235) : {ActionCnt += 1;}
    (junction 235) -> (junction 234)
    (junction 234) -> (junction 261)
    (junction 261) -> (junction 255) [order 1] : /*调用2 */
        | [PaMem_IVI_FLSeatMemSet2 > enMemSet.EN_MemSet_NULL ...
        | &&PaMem_IVI_FLSeatMemSet2 < enMemSet.EN_MemSet_Clean]
    (junction 261) -> (junction 253) [order 2]
    (junction 255) -> (junction 254) : {ActionCnt += 1;}
    (junction 254) -> (junction 253)
    (junction 253) -> (junction 247)
    (junction 247) -> (junction 246) [order 1] : /* 调用3 */
        | [PaMem_IVI_FLSeatMemSet3 > enMemSet.EN_MemSet_NULL ...
        | &&PaMem_IVI_FLSeatMemSet3 < enMemSet.EN_MemSet_Clean]
    (junction 247) -> (junction 251) [order 2]
    (junction 246) -> (junction 245) : {ActionCnt += 1;}
    (junction 245) -> (junction 251)
    (junction 251) -> (junction 264)
    (junction 264) -> (junction 270) [order 1] : /* 存在冲突 */
        | [ActionCnt >= 2]
    (junction 264) -> (junction 269) [order 2] : {ActionFlag = TRUE;}
    (junction 270) -> (junction 268) : {ActionFlag = FALSE;}
    (junction 268) -> (junction 269)
    (junction 269) -> (junction 236)
  state AcquireMemoryButtonReq [parallel]
    settings: executionOrder=2
    state NoButtonConflict
      state FirstButton [parallel]
        settings: executionOrder=1
        (default) -> (junction 71)
        FirstButton -> (junction 71)
        (junction 71) -> (junction 74)
        (junction 74) -> (junction 76) [order 1] : /* 记忆位置1 */
            | [PaMem_IVI_FLSeatMemSet1 == enMemSet.EN_MemSet_Mem]
        (junction 74) -> (junction 80) [order 2]
        (junction 76) -> (junction 78) : {SeatMemBtn = enMemBtn.EN_MemBtn_Set1;}
        (junction 78) -> (junction 80)
        (junction 80) -> (junction 84)
        (junction 84) -> (junction 86) [order 1] : /* 调用位置1 */
            | [PaMem_IVI_FLSeatMemSet1 == enMemSet.EN_MemSet_Call]
        (junction 84) -> (junction 90) [order 2]
        (junction 86) -> (junction 88) : {SeatMemBtn = enMemBtn.EN_MemBtn_Call1;}
        (junction 88) -> (junction 90)
        (junction 90) -> (junction 93)
        (junction 93) -> (junction 95) [commented out] : /* 清除位置1 */
            | [PaMem_IVI_FLSeatMemSet1 == enMemSet.EN_MemSet_Clean]
        (junction 93) -> (junction 99)
        (junction 95) -> (junction 97) [commented out] : {SeatMemBtn = enMemBtn.EN_MemBtn_Clear1;}
        (junction 97) -> (junction 99) [commented out]
        (junction 99) -> (junction 102)
      state SecondButton [parallel]
        settings: executionOrder=2
        (default) -> (junction 105)
        SecondButton -> (junction 105)
        (junction 105) -> (junction 110)
        (junction 110) -> (junction 114) [order 1] : /* 记忆位置2 */
            | [PaMem_IVI_FLSeatMemSet2 == enMemSet.EN_MemSet_Mem]
        (junction 110) -> (junction 117) [order 2]
        (junction 114) -> (junction 119) : {SeatMemBtn = enMemBtn.EN_MemBtn_Set2;}
        (junction 119) -> (junction 117)
        (junction 117) -> (junction 112)
        (junction 112) -> (junction 107) [order 1] : /* 调用位置2 */
            | [PaMem_IVI_FLSeatMemSet2 == enMemSet.EN_MemSet_Call]
        (junction 112) -> (junction 115) [order 2]
        (junction 107) -> (junction 120) : {SeatMemBtn = enMemBtn.EN_MemBtn_Call2;}
        (junction 120) -> (junction 115)
        (junction 115) -> (junction 125)
        (junction 125) -> (junction 126) [commented out] : /* 清除位置2 */
            | [PaMem_IVI_FLSeatMemSet2 == enMemSet.EN_MemSet_Clean]
        (junction 125) -> (junction 108)
        (junction 126) -> (junction 127) [commented out] : {SeatMemBtn = enMemBtn.EN_MemBtn_Clear2;}
        (junction 127) -> (junction 108) [commented out]
        (junction 108) -> (junction 128)
      state ThirdButton [parallel]
        settings: executionOrder=3
        (default) -> (junction 140)
        ThirdButton -> (junction 140)
        (junction 140) -> (junction 141)
        (junction 141) -> (junction 144) [order 1] : /* 记忆位置3 */
            | [PaMem_IVI_FLSeatMemSet3 == enMemSet.EN_MemSet_Mem]
        (junction 141) -> (junction 146) [order 2]
        (junction 144) -> (junction 147) : {SeatMemBtn = enMemBtn.EN_MemBtn_Set3;}
        (junction 147) -> (junction 146)
        (junction 146) -> (junction 150)
        (junction 150) -> (junction 153) [order 1] : /* 调用位置3 */
            | [PaMem_IVI_FLSeatMemSet3 == enMemSet.EN_MemSet_Call]
        (junction 150) -> (junction 155) [order 2]
        (junction 153) -> (junction 158) : {SeatMemBtn = enMemBtn.EN_MemBtn_Call3;}
        (junction 158) -> (junction 155)
        (junction 155) -> (junction 149)
        (junction 149) -> (junction 154) [commented out] : /* 清除位置3 */
            | [PaMem_IVI_FLSeatMemSet3 == enMemSet.EN_MemSet_Clean]
        (junction 149) -> (junction 145)
        (junction 154) -> (junction 138) [commented out] : {SeatMemBtn = enMemBtn.EN_MemBtn_Clear3;}
        (junction 138) -> (junction 145) [commented out]
        (junction 145) -> (junction 156)
      state CleanButtonReq [parallel]
        settings: executionOrder=4
        (default) -> (junction 172)
        CleanButtonReq -> (junction 172)
        (junction 172) -> (junction 175)
        (junction 175) -> (junction 177) [order 1] : /* 无记忆请求 */
            | [PaMem_IVI_FLSeatMemSet1 == enMemSet.EN_MemSet_NULL ...
            | && PaMem_IVI_FLSeatMemSet2 == enMemSet.EN_MemSet_NULL ...
            | && PaMem_IVI_FLSeatMemSet3 == enMemSet.EN_MemSet_NULL]
        (junction 175) -> (junction 181) [order 2]
        (junction 177) -> (junction 179) : {SeatMemBtn = enMemBtn.EN_MemBtn_NULL;}
        (junction 179) -> (junction 181)
        (junction 181) -> (junction 182)
    state ButtonConflict
      en:
      SeatMemBtn = enMemBtn.EN_MemBtn_NULL;
    (default) -> ButtonConflict
    ButtonConflict -> NoButtonConflict : /*无报文冲突*/
        | [ActionFlag == TRUE]
    NoButtonConflict -> ButtonConflict : /*报文冲突*/
        | [ActionFlag == FALSE]
  data: PaMem_IVI_FLSeatMemSet1 input; PaMem_IVI_FLSeatMemSet2 input; SeatMemBtn output Enum: enMemBtn; TRUE parameter; FALSE parameter; PaMem_IVI_FLSeatMemSet3 input; ActionFlag local double; ActionCnt local uint8

== stateflow chart Appl_PaMemory_CtrlModel/UpDataInputInfo/InputSignalProcess/MemorySetCallPreconditionDeal/PreconditionDeal ==
  state MemorySetPreconditionDeal [parallel]
    settings: executionOrder=1
    state PreconditionSatisfied
      en:
      MemSetPC_Flag = TRUE;
    state PreconditionNotSatisfied
      en:
      MemSetPC_Flag = FALSE;
    (default) -> MemorySetPreconditionDeal.PreconditionNotSatisfied
    MemorySetPreconditionDeal.PreconditionNotSatisfied -> MemorySetPreconditionDeal.PreconditionSatisfied : /*副驾驶调节配置==TRUE
        | &&记忆功能使能 == 0x1:TRUE
        | && 座椅已学习
        | && 座椅运动类型 == 0x0:enNULL
        | && 座椅霍尔故障标志位 == FALSE
        | && 座椅继电器粘连故障标志位 == FALSE
        | && 座椅堵转故障标志位 == FALSE
        | && IVI_NapMode_SwtichSet != 0x1:打开小憩模式
        | && 电压模式 == 正常
        | /PreMemSetStop = 0x0:enNone;*/
        | [PaMem_AdjustEnable == TRUE ...
        | && PaMem_PaMemoryConfig == TRUE ...
        | && PaMem_SeatLearnResult == TRUE ...
        | && PaMem_CurrentMoveType == enSeatMotorRunType.EN_NULL ...
        | && PaMem_AnyoneHallFaultSts == FALSE ...
        | && PaMem_AnyoneRelayFaultSts == FALSE ...
        | && PaMem_PaAnyoneLockFaultSts == FALSE ...
        | && PaMem_NapMode != enNapMode.EN_NapMode_Open...
        | && PaMem_VoltSatisfy == TRUE ...
        | && PaMem_VoltMode == enFinalPowerMode.EN_NORMAL_VOLT]
        | /PreMemSetStop = enMemStopCause.EN_MemStop_NULL;
    MemorySetPreconditionDeal.PreconditionSatisfied -> MemorySetPreconditionDeal.PreconditionNotSatisfied [order 1] : /*记忆功能使能 != 0x1:TRUE
        | /PreMemCallStop = 0xA:enConfigError;*/
        | [PaMem_AdjustEnable != TRUE || PaMem_PaMemoryConfig != TRUE ]
        | /PreMemSetStop = enMemStopCause.EN_MemStop_ConfigError;
    MemorySetPreconditionDeal.PreconditionSatisfied -> MemorySetPreconditionDeal.PreconditionNotSatisfied [order 2] : /*!座椅已学习
        | /PreMemSetStop = 0x1:enNotLearn;*/
        | [PaMem_SeatLearnResult != TRUE]
        | /PreMemSetStop = enMemStopCause.EN_MemStop_Learn;
    MemorySetPreconditionDeal.PreconditionSatisfied -> MemorySetPreconditionDeal.PreconditionNotSatisfied [order 3] : /*座椅运动类型 != 0x0:enNULL
        | /PreMemSetStop = 0x2:enOtherMove;*/
        | [PaMem_CurrentMoveType != enSeatMotorRunType.EN_NULL]
        | /PreMemSetStop = enMemStopCause.EN_MemStop_OtherMove;
    MemorySetPreconditionDeal.PreconditionSatisfied -> MemorySetPreconditionDeal.PreconditionNotSatisfied [order 4] : /*座椅霍尔故障标志位 != FALSE
        | /PreMemSetStop = 0x3:enHallError;*/
        | [PaMem_AnyoneHallFaultSts != FALSE]
        | /PreMemSetStop = enMemStopCause.EN_MemStop_HallErr;
    MemorySetPreconditionDeal.PreconditionSatisfied -> MemorySetPreconditionDeal.PreconditionNotSatisfied [order 5] : /*座椅继电器粘连故障标志位 != FALSE
        | /PreMemSetStop = 0x4:enRelayError;*/
        | [PaMem_AnyoneRelayFaultSts != FALSE]
        | /PreMemSetStop = enMemStopCause.EN_MemStop_RelayErr;
    MemorySetPreconditionDeal.PreconditionSatisfied -> MemorySetPreconditionDeal.PreconditionNotSatisfied [order 6] : /*IVI_NapMode_SwtichSet == 0x1:打开小憩模式
        | /PreMemSetStop = 0xB:enNapError;*/
        | [PaMem_NapMode == enNapMode.EN_NapMode_Open]
        | /PreMemSetStop = enMemStopCause.EN_MemStop_NapError;
    MemorySetPreconditionDeal.PreconditionSatisfied -> MemorySetPreconditionDeal.PreconditionNotSatisfied [order 8] : /*座椅堵转故障标志位 != FALSE
        | /PreMemSetStop = 0x:EN_MemStop_StallErr;*/
        | [PaMem_PaAnyoneLockFaultSts != FALSE]
        | /PreMemSetStop = enMemStopCause.EN_MemStop_StallErr;
    MemorySetPreconditionDeal.PreconditionSatisfied -> MemorySetPreconditionDeal.PreconditionNotSatisfied [order 7] : /*电压模式 != 正常
        | /PreMemSetStop = 0xE:enVoltageError;*/
        | [PaMem_VoltMode != enFinalPowerMode.EN_NORMAL_VOLT ...
        | ||  PaMem_VoltSatisfy != TRUE]
        | /PreMemSetStop = enMemStopCause.EN_MemStop_VoltageErr;
  state MemoryCallPreconditionDeal [parallel]
    settings: executionOrder=2
    state PreconditionSatisfied
      en:
      MemCallPC_Flag = TRUE;
    state PreconditionNotSatisfied
      en:
      MemCallPC_Flag = FALSE;
    (default) -> MemoryCallPreconditionDeal.PreconditionNotSatisfied
    MemoryCallPreconditionDeal.PreconditionNotSatisfied -> MemoryCallPreconditionDeal.PreconditionSatisfied : /*副驾驶调节配置==TRUE
        | && 记忆功能使能 == 0x1:TRUE
        | && 电源档位 != 0x3:enCRANK
        | && 座椅已学习
        | && 座椅继电器粘连故障标志位 == FALSE
        | && SpeedLessThan5_Flag == TRUE
        | && 座椅运动类型 <= 0x3:enMemory
        | && 电压模式 == 正常
        | && 座椅按键标志位 == FALSE
        | && DSM_NapMode_FB != 0x2:打开小憩模式
        | /PreMemCallStop = 0x0:enNone;*//*&& PaMem_Gear_PN_FlagOut == TRUE ...*/
        | [PaMem_AdjustEnable == TRUE ...
        | && PaMem_PaMemoryConfig == TRUE ...
        | && PaMem_PowerMode != enPowerModeSts.EN_CRANK ...
        | && PaMem_SeatLearnResult == TRUE ...
        | && PaMem_AnyoneRelayFaultSts == FALSE ...
        | && SpeedLessThan5_Flag == TRUE ...
        | && PaMem_CurrentMoveType <= enSeatMotorRunType.EN_MemoryEnable ...
        | && PaMem_VoltSatisfy == TRUE ...
        | && PaMem_PALengthSwitch == FALSE ...
        | && PaMem_PABackSwitch ==FALSE ...
        | && PaMem_VoltMode == enFinalPowerMode.EN_NORMAL_VOLT ...
        | && PaMem_NapMode != enNapMode.EN_NapMode_Open]
        | /PreMemCallStop = enMemStopCause.EN_MemStop_NULL;
    MemoryCallPreconditionDeal.PreconditionSatisfied -> MemoryCallPreconditionDeal.PreconditionNotSatisfied [order 1] : /*记忆功能使能 != 0x1:TRUE
        | /PreMemCallStop = 0xA:enConfigError;*/
        | [PaMem_AdjustEnable != TRUE || PaMem_PaMemoryConfig != TRUE]
        | /PreMemCallStop = enMemStopCause.EN_MemStop_ConfigError;
    MemoryCallPreconditionDeal.PreconditionSatisfied -> MemoryCallPreconditionDeal.PreconditionNotSatisfied [order 7] : /*电源档位 == 0x3:enCRANK
        | /PreMemCallStop = 0x6:enNotON;*/
        | [PaMem_PowerMode == enPowerModeSts.EN_CRANK]
        | /PreMemCallStop = enMemStopCause.EN_MemStop_NotON;
    MemoryCallPreconditionDeal.PreconditionSatisfied -> MemoryCallPreconditionDeal.PreconditionNotSatisfied [commented out] : /*GearPN_Flag != TRUE
        | /PreMemCallStop = 0x7:enNotGearPN;*/
        | [PaMem_Gear_PN_FlagOut != TRUE]
        | /PreMemCallStop = enMemStopCause.EN_MemStop_NotGearPN;
    MemoryCallPreconditionDeal.PreconditionSatisfied -> MemoryCallPreconditionDeal.PreconditionNotSatisfied [order 2] : /*!座椅已学习
        | /PreMemSetStop = 0x1:enNotLearn;*/
        | [PaMem_SeatLearnResult != TRUE]
        | /PreMemCallStop = enMemStopCause.EN_MemStop_Learn;
    MemoryCallPreconditionDeal.PreconditionSatisfied -> MemoryCallPreconditionDeal.PreconditionNotSatisfied [order 4] : /*座椅继电器粘连故障标志位 != FALSE
        | /PreMemSetStop = 0x4:enRelayError;*/
        | [PaMem_AnyoneRelayFaultSts != FALSE]
        | /PreMemCallStop = enMemStopCause.EN_MemStop_RelayErr;
    MemoryCallPreconditionDeal.PreconditionSatisfied -> MemoryCallPreconditionDeal.PreconditionNotSatisfied [order 8] : /*SpeedLessThan5_Flag != TRUE
        | /PreMemCallStop = 0x8:enSpeedError;*/
        | [SpeedLessThan5_Flag != TRUE]
        | /PreMemCallStop = enMemStopCause.EN_MemStop_SpeedError;
    MemoryCallPreconditionDeal.PreconditionSatisfied -> MemoryCallPreconditionDeal.PreconditionNotSatisfied [order 3] : /*座椅运动类型 > 0x3:enMemory
        | /PreMemCallStop = 0x2:enOtherMove;*/
        | [PaMem_CurrentMoveType > enSeatMotorRunType.EN_MemoryEnable]
        | /PreMemCallStop = enMemStopCause.EN_MemStop_OtherMove;
    MemoryCallPreconditionDeal.PreconditionSatisfied -> MemoryCallPreconditionDeal.PreconditionNotSatisfied [order 5] : /*IVI_NapMode_SwtichSet == 0x1:打开小憩模式
        | /PreMemSetStop = 0xB:enNapError;*/
        | [PaMem_NapMode == enNapMode.EN_NapMode_Open]
        | /PreMemCallStop = enMemStopCause.EN_MemStop_NapError;
    MemoryCallPreconditionDeal.PreconditionSatisfied -> MemoryCallPreconditionDeal.PreconditionNotSatisfied [order 6] : /*电压模式 != 正常
        | /PreMemSetStop = 0xE:enVoltageError;*/
        | [PaMem_VoltMode != enFinalPowerMode.EN_NORMAL_VOLT...
        | ||  PaMem_VoltSatisfy != TRUE]
        | /PreMemCallStop = enMemStopCause.EN_MemStop_VoltageErr;
    MemoryCallPreconditionDeal.PreconditionSatisfied -> MemoryCallPreconditionDeal.PreconditionNotSatisfied [order 9] : /*座椅按键标志位 != FALSE
        | /PreMemSetStop = 0x:EN_MemStop_StallErr;*/
        | [PaMem_PALengthSwitch != FALSE ...
        | || PaMem_PABackSwitch !=FALSE ]
        | /PreMemCallStop = enMemStopCause.EN_MemStop_StallErr;
  data: FALSE parameter; TRUE parameter; PaMem_Gear_PN_FlagOut input; PaMem_PowerMode input; PaMem_VoltMode input; PaMem_AdjustEnable input; PaMem_AnyoneHallFaultSts input; PaMem_AnyoneRelayFaultSts input; PaMem_CurrentMoveType input; PaMem_SeatLearnResult input; PaMem_NapMode input; SpeedLessThan5_Flag input; MemSetPC_Flag output uint8; PreMemSetStop output Enum: enMemStopCause; MemCallPC_Flag output uint8; PreMemCallStop output Enum: enMemStopCause; PaMem_PaMemoryConfig input; PaMem_PaAnyoneLockFaultSts input; PaMem_VoltSatisfy input; PaMem_PAHeightSwitch input; PaMem_PALengthSwitch input; PaMem_PABackSwitch input; PaMem_PAFrontSwitch input
